simulink model "prox_sensor_gen"  (R2018a)
settings: Solver=VariableStepAuto  StartTime=0.0  StopTime=10.0  RelTol=1e-3
settings Model: Creator=blond  LastModifiedBy=blond

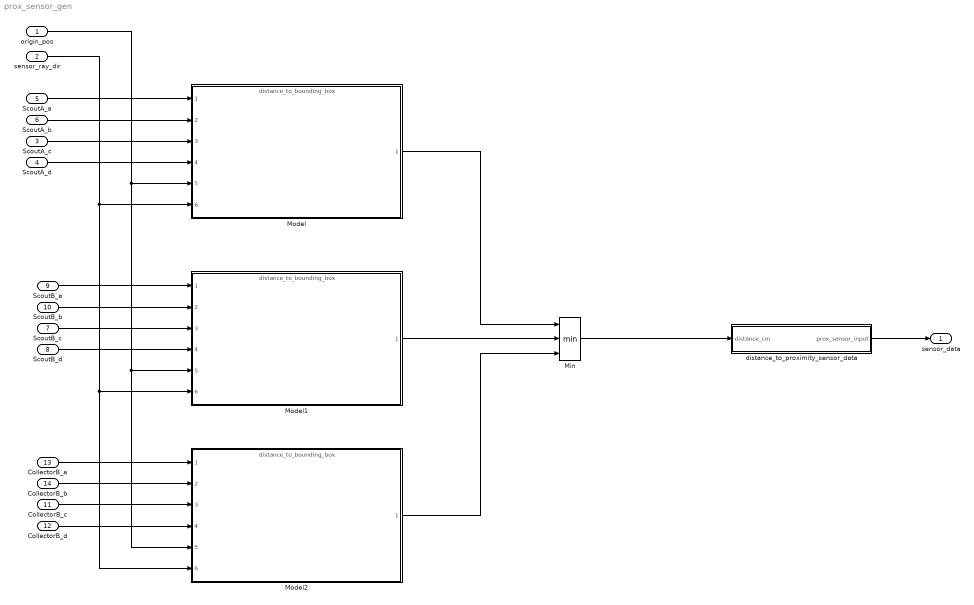
== system prox_sensor_gen ==
  origin_pos : Inport
  sensor_ray_dir : Inport  Port=2
  ScoutA_c : Inport  Port=3
  ScoutA_d : Inport  Port=4
  ScoutA_a : Inport  Port=5
  ScoutA_b : Inport  Port=6
  ScoutB_c : Inport  Port=7
  ScoutB_d : Inport  Port=8
  ScoutB_a : Inport  Port=9
  ScoutB_b : Inport  Port=10
  CollectorB_c : Inport  Port=11
  CollectorB_d : Inport  Port=12
  CollectorB_a : Inport  Port=13
  CollectorB_b : Inport  Port=14
  Min : MinMax  Inputs=3
  Model : ModelReference  ModelNameDialog=distance_to_bounding_box.slx  SimulationMode=Normal  ModelReferenceVersion=1.2
  Model1 : ModelReference  ModelNameDialog=distance_to_bounding_box.slx  SimulationMode=Normal  ModelReferenceVersion=1.2
  Model2 : ModelReference  ModelNameDialog=distance_to_bounding_box.slx  SimulationMode=Normal  ModelReferenceVersion=1.2
  "distance_to_proximity_sensor_data " : Subsystem
  "sensor_data " : Outport
  wires:
  ScoutB_a/1 -> Model1/1
  Model2/1 -> Min/3
  ScoutB_c/1 -> Model1/3
  CollectorB_b/1 -> Model2/2
  CollectorB_d/1 -> Model2/4
  CollectorB_a/1 -> Model2/1
  CollectorB_c/1 -> Model2/3
  ScoutA_a/1 -> Model/1
  ScoutA_c/1 -> Model/3
  Model/1 -> Min/1
  ScoutA_d/1 -> Model/4
  ScoutA_b/1 -> Model/2
  Model1/1 -> Min/2
  ScoutB_b/1 -> Model1/2
  "distance_to_proximity_sensor_data "/1("prox_sensor_input ") -> "sensor_data "/1
  ScoutB_d/1 -> Model1/4
  Min/1 -> "distance_to_proximity_sensor_data "/1(distance_cm)
  origin_pos/1 -> Model/5, Model2/5, Model1/5
  sensor_ray_dir/1 -> Model/6, Model2/6, Model1/6

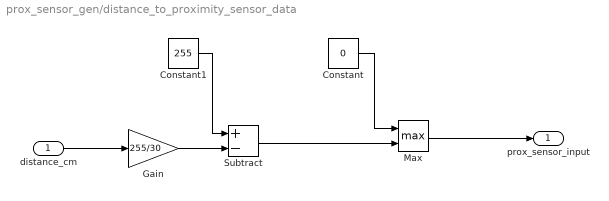
== system prox_sensor_gen/distance_to_proximity_sensor_data  ==
  distance_cm : Inport
  Constant : Constant  Value=0
  Constant1 : Constant  Value=255
  Gain : Gain  Gain=255/30
  Max : MinMax  Function=max  Inputs=2
  Subtract : Sum  Inputs=+-
  "prox_sensor_input " : Outport
  wires:
  distance_cm/1 -> Gain/1
  Gain/1 -> Subtract/2
  Subtract/1 -> Max/2
  Constant/1 -> Max/1
  Max/1 -> "prox_sensor_input "/1
  Constant1/1 -> Subtract/1
